simulink model "position_model_group12"  (R2014a)
settings: Solver=ode45  StartTime=0.0  StopTime=30  RelTol=1e-3
undefined symbols (not defined in the file): ts
libraries: simulink x2
settings Model: Creator=zeinab  LastModifiedBy=zeinab

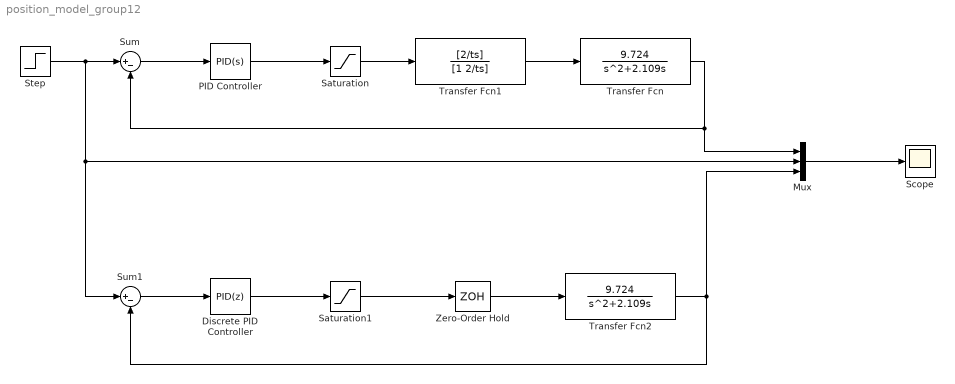
== system position_model_group12 ==
  Discrete PID Controller : simulink/Continuous/PID Controller  Controller=PID  TimeDomain=Discrete-time  SampleTime=ts  IntegratorMethod=Trapezoidal  FilterMethod=Trapezoidal  Form=Parallel  P=0.352639204196396  I=0.0105365075291842  D=0.152688812283356  N=6.17778105040572  InitialConditionSource=internal  InitialConditionForIntegrator=0  InitialConditionForFilter=0  ExternalReset=none  LimitOutput=off  UpperSaturationLimit=inf  LowerSaturationLimit=-inf  LinearizeAsGain=off  AntiWindupMode=none  Kb=1  TrackingMode=off  Kt=1  PParamMin=[]  PParamMax=[]  IParamMin=[]  IParamMax=[]  DParamMin=[]  DParamMax=[]  NParamMin=[]  NParamMax=[]  KbParamMin=[]  KbParamMax=[]  KtParamMin=[]  KtParamMax=[]  POutMin=[]  POutMax=[]  IOutMin=[]  IOutMax=[]  DOutMin=[]  DOutMax=[]  NOutMin=[]  NOutMax=[]  KbOutMin=[]  KbOutMax=[]  KtOutMin=[]  KtOutMax=[]  IntegratorOutMin=[]  IntegratorOutMax=[]  FilterOutMin=[]  FilterOutMax=[]  SumOutMin=[]  SumOutMax=[]  SumI1OutMin=[]  SumI1OutMax=[]  SumI2OutMin=[]  SumI2OutMax=[]  SumI3OutMin=[]  SumI3OutMax=[]  SumDOutMin=[]  SumDOutMax=[]  SaturationOutMin=[]  SaturationOutMax=[]  IntegratorContinuousStateAttributes=''  IntegratorStateMustResolveToSignalObject=off  IntegratorRTWStateStorageClass=Auto  FilterContinuousStateAttributes=''  FilterStateMustResolveToSignalObject=off  FilterRTWStateStorageClass=Auto
  Mux : Mux  Inputs=3
  PID Controller : simulink/Continuous/PID Controller  Controller=PID  TimeDomain=Continuous-time  SampleTime=1  IntegratorMethod=Forward Euler  FilterMethod=Forward Euler  Form=Parallel  P=0.352639204196396  I=0.0105365075291842  D=0.152688812283356  N=6.17778105040572  InitialConditionSource=internal  InitialConditionForIntegrator=0  InitialConditionForFilter=0  ExternalReset=none  LimitOutput=off  UpperSaturationLimit=inf  LowerSaturationLimit=-inf  LinearizeAsGain=on  AntiWindupMode=none  Kb=1  TrackingMode=off  Kt=1  PParamMin=[]  PParamMax=[]  IParamMin=[]  IParamMax=[]  DParamMin=[]  DParamMax=[]  NParamMin=[]  NParamMax=[]  KbParamMin=[]  KbParamMax=[]  KtParamMin=[]  KtParamMax=[]  POutMin=[]  POutMax=[]  IOutMin=[]  IOutMax=[]  DOutMin=[]  DOutMax=[]  NOutMin=[]  NOutMax=[]  KbOutMin=[]  KbOutMax=[]  KtOutMin=[]  KtOutMax=[]  IntegratorOutMin=[]  IntegratorOutMax=[]  FilterOutMin=[]  FilterOutMax=[]  SumOutMin=[]  SumOutMax=[]  SumI1OutMin=[]  SumI1OutMax=[]  SumI2OutMin=[]  SumI2OutMax=[]  SumI3OutMin=[]  SumI3OutMax=[]  SumDOutMin=[]  SumDOutMax=[]  SaturationOutMin=[]  SaturationOutMax=[]  IntegratorContinuousStateAttributes=''  IntegratorStateMustResolveToSignalObject=off  IntegratorRTWStateStorageClass=Auto  FilterContinuousStateAttributes=''  FilterStateMustResolveToSignalObject=off  FilterRTWStateStorageClass=Auto
  Saturation : Saturate  UpperLimit=6  LowerLimit=-6  SampleTime=ts
  Saturation1 : Saturate  UpperLimit=6  LowerLimit=-6  SampleTime=ts
  Scope : Scope
      settings: YMin=0  YMax=1.75
  Step : Step  After=0.5*3.14  SampleTime=ts
  Sum : Sum  Inputs=|+-
  Sum1 : Sum  Inputs=|+-
  Transfer Fcn : TransferFcn  Numerator=[9.724]  Denominator=[1 2.109 0]
  Transfer Fcn1 : TransferFcn  Numerator=[2/ts]  Denominator=[1 2/ts]
  Transfer Fcn2 : TransferFcn  Numerator=[9.724]  Denominator=[1 2.109 0]
  Zero-Order Hold : ZeroOrderHold  SampleTime=ts
  wires:
  Transfer Fcn1/1 -> Transfer Fcn/1
  PID Controller/1 -> Saturation/1
  Sum/1 -> PID Controller/1
  Transfer Fcn/1 -> Mux/1, Sum/2
  Step/1 -> Sum1/1, Mux/2, Sum/1
  Mux/1 -> Scope/1
  Saturation/1 -> Transfer Fcn1/1
  Zero-Order Hold/1 -> Transfer Fcn2/1
  Saturation1/1 -> Zero-Order Hold/1
  Discrete PID Controller/1 -> Saturation1/1
  Sum1/1 -> Discrete PID Controller/1
  Transfer Fcn2/1 -> Mux/3, Sum1/2
